simulink library "NonlinearModel_Lib"  (Simulink 7.5)
settings: Solver=ode45  StartTime=0.0  StopTime=10.0  RelTol=1e-3
values from neighbouring files (symbols this model uses):
  AC = FASER_config    [UAV_config.m]    (also in UAV_modelconfig.mat = )
  TrimCondition =     [UAV_trimcondition.mat]
undefined symbols (not defined in the file or in its folder): m, s
libraries: simulink x3, aerolib6dofsys x3, aerolibconvert2 x2, aerolibutil x1, AuxEq_Lib x1, Environment_Lib x1, Aero_Lib x1, Propulsion_Lib x1, Gravity_Lib x1
settings Model: Creator=Paul Freeman  LastModifiedBy=austinmurch

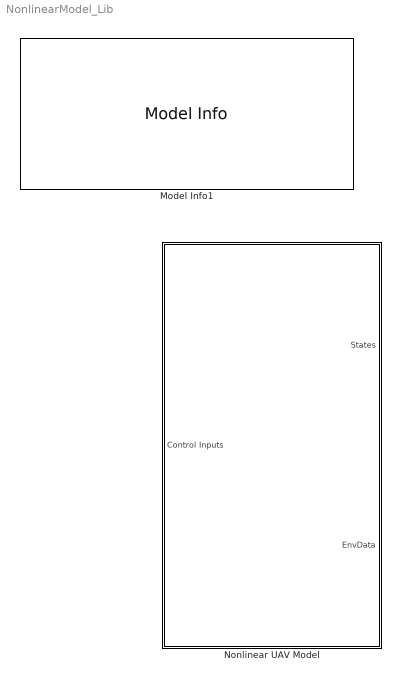
== system NonlinearModel_Lib ==
  Model Info1 : simulink/Model-Wide Utilities/Model Info  SystemSampleTime=-1  InitialBlockCM=None  BlockCM=None  Frame=on  DisplayStringWithTags=|  HorizontalTextAlignment=Left  LeftAlignmentValue=0.02  SourceBlockDiagram=NonlinearModel_Lib  TagMaxNumber=20
      | MODEL INFORMATION
      | UAV Nonlinear Model Library
      | 
      | University of Minnesota
      | Aerospace Engineering and Mechanics
      | Copyright 2011 Regents of the University of Minnesota. All rights reserved.
      | 
      | == SVN Info ==
      | %<ModelVersion>
      | Last modified by %<LastModifiedBy> on %<LastModificationDate>
  Nonlinear UAV Model : Subsystem

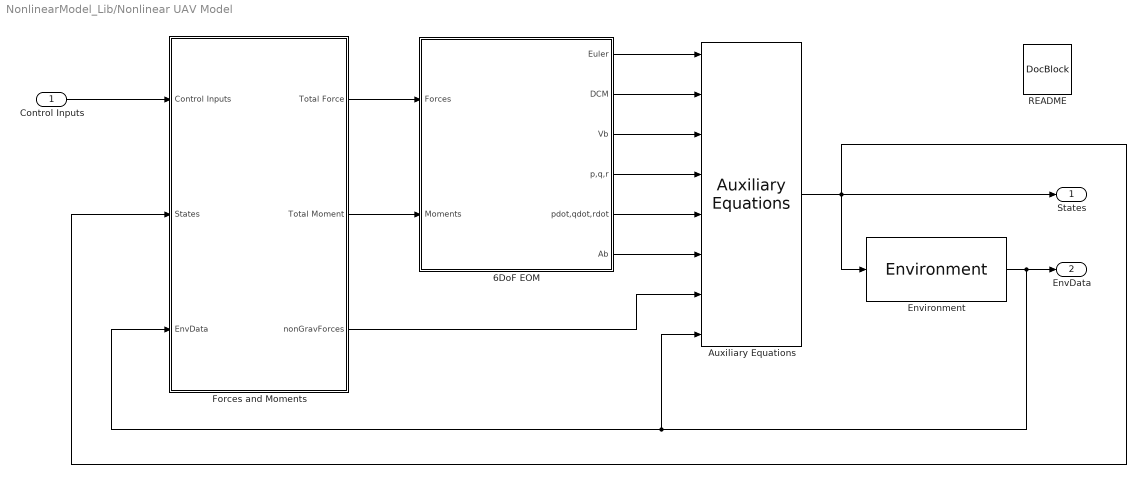
== system NonlinearModel_Lib/Nonlinear UAV Model ==
  Control Inputs : Inport
  6DoF EOM : Subsystem  mask(6DoF EoM (Body Axis)){units=Metric (MKS), mtype=Fixed, rep=Euler Angles, xme_0=TrimCondition.InertialIni, Vm_0=TrimCondition.VelocitiesIni, eul_0=TrimCondition.AttitudeIni, pm_0=TrimCondition.RatesIni, mass_0=AC.Mass, mass_e=0.5, mass_f=2.0, inertia=AC.Inertia.Matrix, inertia_e=eye(3), inertia_f=2*eye(3), k_quat=1.0}
      mask prompts: mtype "Mass type:"; rep "Representation:"; xme_0 "Initial position in inertial axes [Xe,Ye,Ze]:"; Vm_0 "Initial velocity in body axes [U,v,w]:"; eul_0 "Initial Euler orientation [roll, pitch, yaw]:"; pm_0 "Initial body rotation rates [p,q,r]:"; mass_0 "Initial mass:"; mass_e "Empty mass:"; mass_f "Full mass:"; inertia_e "Empty inertia matrix:"; inertia_f "Full inertia matrix:"; k_quat "Gain for quaternion normalization:"
      mask help:
      | Integrate the six-degrees-of-freedom equations of motion in body axis.
      |
      | This block has been modified from the original Aerospace Blockset
      | implementation. The inertial position vector (Xe) is no longer computed.
      | The original block did not have a way to add steady state winds to the
      | inertial velocities (Ve) prior to integrating to get Xe. Therefore, this
      | step is performed in the Auxiliary Equations block.
      mask Help: eval('asbhelp(''sixdof_euler_angles'')');
      mask StyleString: popup(Metric (MKS)|English (Velocity in ft/s)|English (Velocity in kts)),popup(Fixed|Simple Variable|Custom Variable),popup(Euler Angles|Quaternion),edit,edit,edit,edit,edit,edit,edit,edit,edit,edit,edit
      mask CallbackString: |aeroicon('aeroblk6dofbody');|aeroicon('aeroblk6dofbody');|||||||||||
  Auxiliary Equations : AuxEq_Lib/Auxiliary Equations  SystemSampleTime=-1
  Environment : Environment_Lib/Environment  SystemSampleTime=-1
  Forces and Moments : Subsystem
  README : simulink/Model-Wide Utilities/DocBlock  SystemSampleTime=-1  DocumentType=Text
  States : Outport  OutDataType=sfix(16)  OutScaling=2^0
  EnvData : Outport  Port=2  OutDataType=sfix(16)  OutScaling=2^0
  wires:
  Environment/1 -> EnvData/1, Auxiliary Equations/8, Forces and Moments/3(EnvData)
  Forces and Moments/3(nonGravForces) -> Auxiliary Equations/7
  Auxiliary Equations/1 -> Forces and Moments/2(States), Environment/1, States/1
  Forces and Moments/2(Total Moment) -> 6DoF EOM/2(Moments)
  Forces and Moments/1(Total Force) -> 6DoF EOM/1(Forces)
  Control Inputs/1 -> Forces and Moments/1(Control Inputs)
  6DoF EOM/1(Euler) -> Auxiliary Equations/1
  6DoF EOM/2(DCM) -> Auxiliary Equations/2
  6DoF EOM/3(Vb) -> Auxiliary Equations/3
  6DoF EOM/4(p,q,r) -> Auxiliary Equations/4
  6DoF EOM/5(pdot,qdot,rdot) -> Auxiliary Equations/5
  6DoF EOM/6(Ab) -> Auxiliary Equations/6

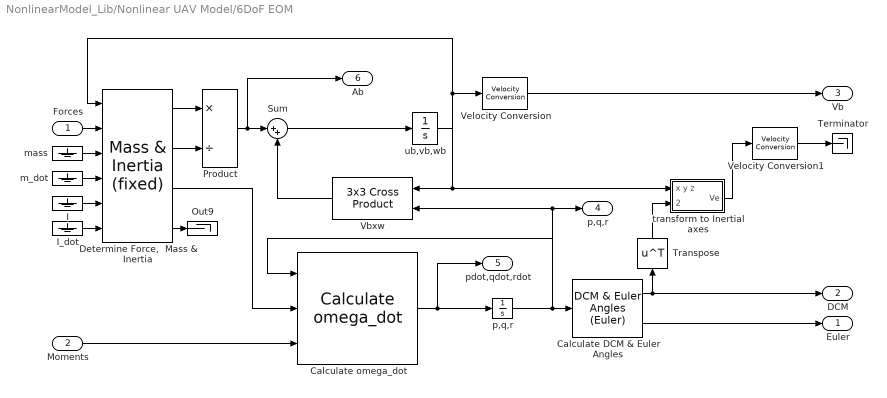
== system NonlinearModel_Lib/Nonlinear UAV Model/6DoF EOM ==
  Forces : Inport  OutDataType=sfix(16)  OutScaling=2^0
  Moments : Inport  Port=2  OutDataType=sfix(16)  OutScaling=2^0
  Calculate DCM & Euler Angles : aerolib6dofsys/DCM & Euler Angles (Euler)  SystemSampleTime=-1
  Calculate omega_dot : aerolib6dofsys/Calculate omega_dot  SystemSampleTime=-1
  "Determine Force,  Mass & Inertia" : aerolib6dofsys/Mass & Inertia (fixed)  SystemSampleTime=-1
  I : Ground
  I_dot : Ground
  Out9 : Terminator
  Product : Product  Inputs=*/  OutDataType=sfix(16)  OutScaling=2^0  SaturateOnIntegerOverflow=on  OutDataTypeStr=Inherit: Same as first input
  Sum : Sum  Inputs=|++  OutDataType=sfix(16)  OutScaling=2^0  SaturateOnIntegerOverflow=on
  Terminator : Terminator
  Transpose : Math  Operator=transpose  OutDataType=sfix(16)  OutScaling=2^0  SaturateOnIntegerOverflow=on
  Vbxw : aerolibutil/3x3 Cross Product  SystemSampleTime=-1
  Velocity Conversion : aerolibconvert2/Velocity Conversion  SystemSampleTime=-1  IU=m/s  OU=m/s
  Velocity Conversion1 : aerolibconvert2/Velocity Conversion  SystemSampleTime=-1  IU=m/s  OU=m/s
  m_dot : Ground
  mass : Ground
  "p,q,r " : Integrator  InitialCondition=pm_0
  "transform to Inertial axes " : Subsystem
      mask Type: Vector Transformation
      mask Display: disp('L_EB')
  ub,vb,wb : Integrator  InitialCondition=convvel(Vm_0,'m/s','m/s')
  Euler : Outport  OutDataType=sfix(16)  OutScaling=2^0
  DCM : Outport  Port=2  OutDataType=sfix(16)  OutScaling=2^0
  Vb : Outport  Port=3  OutDataType=sfix(16)  OutScaling=2^0
  p,q,r : Outport  Port=4  OutDataType=sfix(16)  OutScaling=2^0
  pdot,qdot,rdot : Outport  Port=5  OutDataType=sfix(16)  OutScaling=2^0
  Ab : Outport  Port=6  OutDataType=sfix(16)  OutScaling=2^0
  wires:
  "Determine Force,  Mass & Inertia"/1 -> Product/1
  I_dot/1 -> "Determine Force,  Mass & Inertia"/6
  I/1 -> "Determine Force,  Mass & Inertia"/5
  Calculate omega_dot/1 -> "p,q,r "/1, pdot,qdot,rdot/1
  "Determine Force,  Mass & Inertia"/4 -> Out9/1
  m_dot/1 -> "Determine Force,  Mass & Inertia"/4
  "Determine Force,  Mass & Inertia"/2 -> Product/2
  mass/1 -> "Determine Force,  Mass & Inertia"/3
  Transpose/1 -> "transform to Inertial axes "/2(transform coefficients)
  Calculate DCM & Euler Angles/1 -> Transpose/1, DCM/1
  Product/1 -> Ab/1, Sum/1
  Forces/1 -> "Determine Force,  Mass & Inertia"/2
  Moments/1 -> Calculate omega_dot/3
  "p,q,r "/1 -> Calculate omega_dot/1, Calculate DCM & Euler Angles/1, Vbxw/2, p,q,r/1
  "transform to Inertial axes "/1(Ve) -> Velocity Conversion1/1
  Sum/1 -> ub,vb,wb/1
  ub,vb,wb/1 -> "Determine Force,  Mass & Inertia"/1, Vbxw/1, "transform to Inertial axes "/1(x y z), Velocity Conversion/1
  Vbxw/1 -> Sum/2
  Calculate DCM & Euler Angles/2 -> Euler/1
  "Determine Force,  Mass & Inertia"/3 -> Calculate omega_dot/2
  Velocity Conversion/1 -> Vb/1
  Velocity Conversion1/1 -> Terminator/1

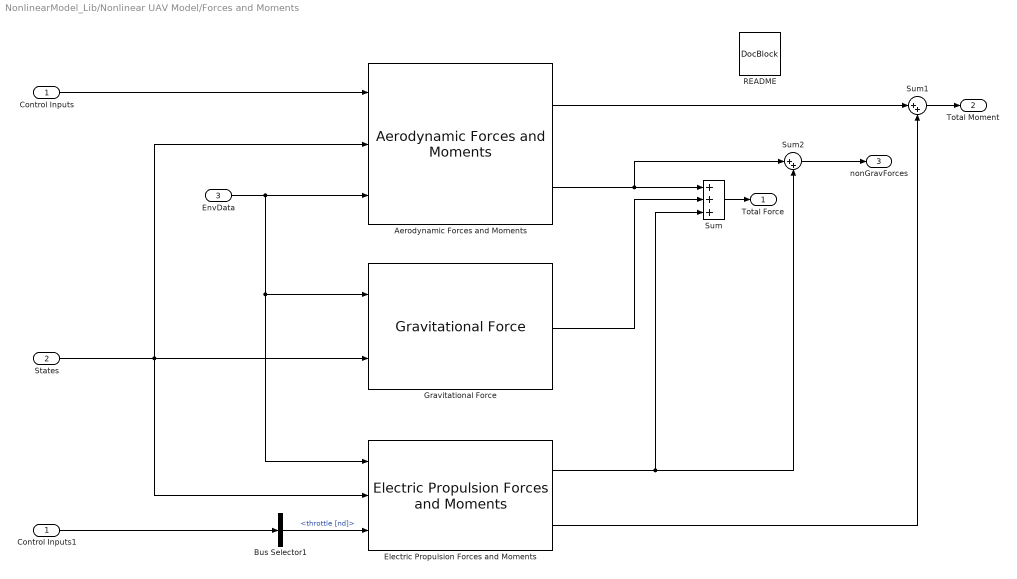
== system NonlinearModel_Lib/Nonlinear UAV Model/Forces and Moments ==
  Control Inputs : Inport
  States : Inport  Port=2
  EnvData : Inport  Port=3
  Aerodynamic Forces and Moments : Aero_Lib/Aerodynamic Forces and Moments  SystemSampleTime=-1  aeromodel=AC.Aero.use_FASER_aero
  Bus Selector1 : BusSelector  OutputSignals=throttle [nd]
  Control Inputs1 : InportShadow  Port=1
  Electric Propulsion Forces and Moments : Propulsion_Lib/Electric Propulsion Forces and Moments  SystemSampleTime=-1
  "Gravitational Force " : Gravity_Lib/Gravitational Force   SystemSampleTime=-1
  README : simulink/Model-Wide Utilities/DocBlock  SystemSampleTime=-1  DocumentType=Text
      content=|
      | Forces and Moments
      |
      | This block models all of the relevant external forces and
      | moments acting on the aircraft. The Aerodynamic Forces and Moments block
      | contains the aero models, and is a masked subsystem. The input parameter to
      | this block is a boolean which controls which aero model (either FASER or
      | the Ultrastick) is used.
      |
      | The Gravitational Force block models the effect of Earth's graviy field on
      | the aircraft.
      |
      | The Electric Propulsion Forces and Moments block contains the electric
      | motor model.
      |
      | Note the non-gravitational forces (nonGravForces) are output- this is what
      | an accelerometer on the aircraft would measure, and is used in the sensor
      | models.
  Sum : Sum  Inputs=+++  OutDataType=sfix(16)  OutScaling=2^0
  Sum1 : Sum  Inputs=|++  OutDataType=sfix(16)  OutScaling=2^0
  Sum2 : Sum  Inputs=|++  OutDataType=fixdt(1, 16)  OutScaling=2^0
  Total Force : Outport
  Total Moment : Outport  Port=2
  nonGravForces : Outport  Port=3
  wires:
  Sum2/1 -> nonGravForces/1
  Sum1/1 -> Total Moment/1
  Electric Propulsion Forces and Moments/2 -> Sum1/2
  Aerodynamic Forces and Moments/1 -> Sum1/1
  Sum/1 -> Total Force/1
  Electric Propulsion Forces and Moments/1 -> Sum/3, Sum2/2
  "Gravitational Force "/1 -> Sum/2
  Aerodynamic Forces and Moments/2 -> Sum2/1, Sum/1
  Control Inputs1/1 -> Bus Selector1/1
  EnvData/1 -> Electric Propulsion Forces and Moments/1, "Gravitational Force "/1, Aerodynamic Forces and Moments/3
  States/1 -> Electric Propulsion Forces and Moments/2, "Gravitational Force "/2, Aerodynamic Forces and Moments/2
  Control Inputs/1 -> Aerodynamic Forces and Moments/1
  Bus Selector1/1 -> Electric Propulsion Forces and Moments/3  "<throttle [nd]>"

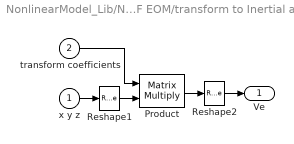
== system NonlinearModel_Lib/Nonlinear UAV Model/6DoF EOM/transform to Inertial axes  ==
  x y z : Inport  OutDataType=sfix(16)  OutScaling=2^0
  transform coefficients : Inport  Port=2  OutDataType=sfix(16)  OutScaling=2^0
  Product : Product  Multiplication=Matrix(*)  OutDataType=sfix(16)  OutScaling=2^0  SaturateOnIntegerOverflow=on  InputSameDT=on  OutDataTypeStr=Inherit: Same as first input
  Reshape1 : Reshape  OutputDimensionality=Column vector (2-D)
  Reshape2 : Reshape
  Ve : Outport  OutDataType=sfix(16)  OutScaling=2^0
  wires:
  Reshape2/1 -> Ve/1
  Reshape1/1 -> Product/2
  x y z/1 -> Reshape1/1
  transform coefficients/1 -> Product/1
  Product/1 -> Reshape2/1
